simulink model "Transm_Ptbs_V1_MkSfunc"  (R2018b)
settings: Solver=ode3  StartTime=0.0  StopTime=660  FixedStep=0.001  RelTol=1e-3
PreLoadFcn:
  | Transm_Ptbs_V1_BusInfo
model workspace (MAT data in the model file):
  DiffRatio = 3.421
  EV_current = 200
  EV_motion = [20 4 0.8]
  EV_sf = 2000
  EngDriveRatio = 0.813008130081
  Fs = 0
  Fv = 0.0025
  Jcomp = 0.0227
  Jengine = 0.22
  Ki = 251.3274
  Kisa = 346.6583
  Kp_d = 0.47149
  Kp_q = 0.52125
  Ksa = 85.4316
  Ksf = 1996.2651
  Ld = 0.0003752
  Ldq = [0.0003752 0.0004148]
  Lq = 0.0004148
  Mechanical = [0.0227 0.0025 0]
  MotGbRatio = 1
  P = 4
  PolePairs = 4
  RWheel = 0.3
  Rs = 0.2
  T_max = 120
  T_mtpa = [0 13.3131834767 26.6278836885 39.9456159322 53.2678926341 66.5962219318 79.9321062746 93.277041051 106.632513247 120.000000141]
  b_axle = Simulink.Parameter
  b_axle.Value = 10
  b_axle.DataType = 'auto'
  b_axle.Dimensions = [1 1]
  b_driveshaft = Simulink.Parameter
  b_driveshaft.Value = 10
  b_driveshaft.DataType = 'auto'
  b_driveshaft.Dimensions = [1 1]
  ba = 3.4029
  id_mtpa = [0 -0.114523352646 -0.457989076459 -1.03008464374 -1.83029075221 -2.85788367342 -4.11193850568 -5.59133329791 -7.29475400168 -9.22070020138]
  idq0 = [0 0]
  idq_limits = [-9.220699542 166.993501392 167.247872355]
  iq_mtpa = [0 18.5827440345 37.1633719111 55.7397734896 74.3098506185 92.871523015 111.422734008 129.961456105 148.485696337 166.993501356]
  k_axle = Simulink.Parameter
  k_axle.Value = 5000
  k_axle.DataType = 'auto'
  k_axle.Dimensions = [1 1]
  k_driveshaft = Simulink.Parameter
  k_driveshaft.Value = 1000
  k_driveshaft.DataType = 'auto'
  k_driveshaft.Dimensions = [1 1]
  lambda_pm = 0.1194
  mechanical = [0.0227 0.0025 0]
  mot.max_trq = 307
  mot.max_pwr = 124
  mot.spd = [0 500 1000 1500 2000 2500 3000 3500 3857.04487493 4000 4500 5000 5500 6000 6500 7000 7500 8000 8500 9000 9500 10000 10500 11000 11500 12000 12500]
  mot.trq = [307 307 307 307 307 307 307 307 307 296.028194151 263.136172579 236.822555321 215.29323211 197.352129434 182.171196401 169.158968086 157.881703547 148.014097075 139.307385483 131.568086289 124.643450169 118.41127766 112.772645391 107.646616055 102.9663284 98.676064717 94.7290221283]
  mot.trq_cp = [296.028194151 263.136172579 236.822555321 215.29323211 197.352129434 182.171196401 169.158968086 157.881703547 148.014097075 139.307385483 131.568086289 124.643450169 118.41127766 112.772645391 107.646616055 102.9663284 98.676064717 94.7290221283]
  mot.J = 0.02
  mot.damp = 0.0001
  mot.Tc = 0.0267
  mot.map.spdindex = [0 1000 2000 3000 3857 4000 5000 6000 7000 8000 9000 10000 11000 12000 12584]
  mot.map.trqindex = [10 25 50 75 100 125 150 175 200 225 250 275 300 307]
  mot.map.eff = [84  90  90  90  90  90  90  90  90  90  90  90  90  90  90; 84  90  93  95  95  95  96  95  95  95  95  93  93  93  93; 84  90  93  95  95  95  96  95  96  95  95  95  95  93  93; 84  90  93  95  95  95  96  96  96  95  95  95  95  93  93; 84  90  93  95  95  95  96  96  96  95  95  93  93  93  90; 84  88  90  93  93  95  95  96  95  95  95  93  93  93  90; 84  88  90  90  90  93  95  95  95  93  93  93  93  93  90; 84  88  90  90  90  90  93  93  93  93  93  93  93  93  90; 84  84  88  90  90  90  93  93  93  93  93  93  93  93  90; 84  84  88  90  90  90  90  93  93  93  93  93  93  93  90; 84  84  84  90  90  90  90  93  93  93  93  93  93  93  90; 84  84  84  88  90  90  90  93  93  93  93  93  93  93  90; 84  84  84  88  88  88  90  93  93  93  93  93  93  93  90; 84  84  84  88  88  88  90  93  93  93  93  93  93  93  90]
  mot.m = 30
  mot.Cp = 200
  omega_init = 0
  theta_init = 0
  wc_shaft = Simulink.Parameter
  wc_shaft.Value = 0.1
  wc_shaft.DataType = 'auto'
  wc_shaft.Dimensions = [1 1]
libraries: autolibtransamt x1
settings Model: Creator=IAEC Nishito  LastModifiedBy=E00026
settings ConfigSet: Description=|
  | プラント、トップモデル用Configurationパラメータ
  | MILS用　固定ステップ
  | Vehicle Network toolbox のCAN通信を、Simulink Desktop Real timeでリアルタイム動作する
settings DataIOCC: SaveFormat=Array  SaveOutput=off  SignalLogging=off  DSMLogging=off  SaveTime=off
settings OptimizationCC: EfficientMapNaN2IntZero=off
settings DebuggingCC: AlgebraicLoopMsg=error  StateNameClashWarn=warning  SFUnexpectedBacktrackingDiag=warning  SFNoUnconditionalDefaultTransitionDiag=warning  SFExecutionAtInitializationDiag=none
settings HardwareCC: ProdBitPerPointer=32  ProdBitPerSizeT=32  ProdBitPerPtrDiffT=32  ProdLargestAtomicFloat=None  ProdIntDivRoundTo=Undefined  ProdEndianess=Unspecified  ProdWordSize=32  ProdHWDeviceType=32-bit Generic  TargetBitPerPointer=64  TargetBitPerSizeT=64  TargetBitPerPtrDiffT=64  TargetLongLongMode=on  TargetIntDivRoundTo=Zero  TargetEndianess=LittleEndian  TargetWordSize=64  TargetHWDeviceType=MATLAB Host  ProdEqTarget=off
settings ModelReferenceCC: PropagateSignalLabelsOutOfModel=off
settings SFSimCC: SimUseLocalCustomCode=off
settings RTWCC: SystemTargetFile=rtwsfcn.tlc  TemplateMakefile=rtwsfcn_default_tmf  Description=S-Function Target  RTWUseLocalCustomCode=off
settings CodeAppCC: MaxIdLength=128
settings STFCustomTargetCC: ModelReferenceCompliant=off  CompOptLevelCompliant=on  MATLABClassNameForMDSCustomization=Simulink.SoftwareTarget.TargetSpecificTriggerConfigurationBase  GRTInterface=on  SystemTargetFile=rtwsfcn.tlc

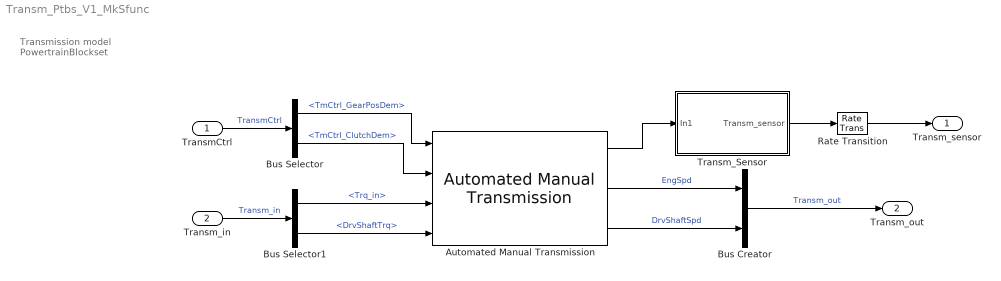
== system Transm_Ptbs_V1_MkSfunc ==
  note: Transmission model
      | PowertrainBlockset
  TransmCtrl : Inport  OutDataTypeStr=Bus: TransmCtrl_Bus  SampleTime=0.001
      settings: AttributesFormatString=|
      | %<OutDataTypeStr>
      | <SampleTime=%<SampleTime>>
  Transm_in : Inport  Port=2  OutDataTypeStr=Bus: Transm_in_Bus  SampleTime=0
      settings: AttributesFormatString=%<OutDataTypeStr>
  Automated Manual Transmission : autolibtransamt/Automated Manual Transmission  VariantControl=0  cntrlType=External control  TransEffModelPopup=Gear only  Jin=.3  bin=.03  omegain_o=0  G=[-1, 0, 1, 2, 3, 4, 5]  Trq_bpts=[25, 50, 75, 100, 150, 200, 250]  omega_bpts=[52.4 78.5 105 131 157 183 209 262 314 419 524]  Temp_bpts=[313 358]  N=[-4.47 ,1, 4.47, 2.47, 1.47, 1, 0.8]  Jout=[0.128 0.01 0.128 0.1 0.062 0.028 0.01]  bout=[.003 .001 .003 .0025 .002 .001 .001]  eta=[0.9, 0.9, 0.9, 0.9, 0.9, 0.95, 0.95]  eta_tbl=reshape([0.53 0.71 0.77 0.79 0.82 0.82 0.82 0.5 0.7 0.77 0.79 0.82 0.82 0.82 0.54 0.72 0.78 0.81 0.83 0.82 0.82 0.56 0.73 0.79 0.81 0.84 0.82 0.82 0.58 0.74 0.79 0.82 0.84 0.82 0.82 0.57 0.74 0.79 0.82 0.84 0.82 0.82 0.58 0.74 0.79 0.82 0.84 0.82 0.82 0.58 0.74 0.79 0.82 0.84 0.82 0.82 0.57 0.74 0.8 0.82 0.85 0.82 0.82 0.55 0.73 0.78 0.81 0.84 0.82 0.82 0.51 0.71 0.77 0.81 0.84 0.82 0.82 0.53 0.71 0.77 0.79 0.82 0.82 0.82 0.5 0.7 0.77 0.79 0.82 0.82 0.82 0.54 0.72 0.78 0.81 0.83 0.82 0.82 0.56 0.73 0.79 0.81 0.84 0.82 0.82 0.58 0.74 0.79 0.82 0.84 0.82 0.82 0.57 0.74 0.79 0.82 0.84 0.82 0.82 0.58 0.74 0.79 0.82 0.84 0.82 0.82 0.58 0.74 0.79 0.82 0.84 0.82 0.82 0.57 0.74 0.8 0.82 0.85 0.82 0.82 0.55 0.73 0.78 0.81 0.84 0.82 0.82 0.51 0.71 0.77 0.81 0.84 0.82 0.82 0.53 0.71 0.77 0.79 0.82 0.82 0.82 0.5 0.7 0.77 0.79 0.82 0.82 0.82 0.54 0.72 0.78 0.81 0.83 0.82 0.82 0.56 0.73 0.79 0.81 0.84 0.82 0.82 0.58 0.74 0.79 0.82 0.84 0.82 0.82 0.57 0.74 0.79 0.82 0.84 0.82 0.82 0.58 0.74 0.79 0.82 0.84 0.82 0.82 0.58 0.74 0.79 0.82 0.84 0.82 0.82 0.57 0.74 0.8 0.82 0.85 0.82 0.82 0.55 0.73 0.78 0.81 0.84 0.82 0.82 0.51 0.71 0.77 0.81 0.84 0.82 0.82 0.7 0.79 0.82 0.83 0.84 0.84 0.84 0.63 0.76 0.8 0.82 0.83 0.84 0.84 0.58 0.74 0.79 0.81 0.83 0.84 0.84 0.58 0.74 0.79 0.81 0.83 0.84 0.84 0.58 0.74 0.79 0.81 0.84 0.84 0.84 0.57 0.73 0.78 0.81 0.84 0.85 0.84 0.57 0.73 0.79 0.81 0.84 0.85 0.84 0.56 0.73 0.78 0.81 0.83 0.85 0.84 0.55 0.73 0.78 0.81 0.84 0.85 0.84 0.52 0.71 0.77 0.8 0.83 0.85 0.84 0.48 0.69 0.76 0.79 0.83 0.84 0.84 0.64 0.76 0.8 0.81 0.83 0.84 0.84 0.56 0.73 0.78 0.8 0.83 0.84 0.84 0.54 0.71 0.77 0.8 0.82 0.84 0.84 0.53 0.71 0.77 0.8 0.83 0.84 0.84 0.51 0.71 0.77 0.8 0.83 0.84 0.85 0.52 0.7 0.77 0.8 0.83 0.84 0.85 0.51 0.71 0.76 0.79 0.83 0.84 0.85 0.5 0.69 0.76 0.79 0.82 0.84 0.85 0.45 0.68 0.75 0.78 0.82 0.84 0.85 0.43 0.67 0.74 0.78 0.81 0.83 0.84 0.38 0.63 0.71 0.75 0.8 0.82 0.83 0.65 0.79 0.84 0.85 0.88 0.89 0.89 0.56 0.75 0.81 0.83 0.86 0.88 0.89 0.52 0.72 0.79 0.83 0.86 0.88 0.88 0.51 0.72 0.79 0.83 0.86 0.88 0.89 0.49 0.71 0.78 0.82 0.86 0.88 0.89 0.47 0.7 0.78 0.82 0.86 0.87 0.88 0.45 0.69 0.77 0.81 0.85 0.87 0.88 0.4 0.67 0.75 0.8 0.84 0.86 0.88 0.3 0.64 0.73 0.78 0.83 0.86 0.87 0.17 0.55 0.67 0.73 0.8 0.83 0.85 0.089 0.45 0.61 0.69 0.77 0.81 0.83 0.61 0.75 0.82 0.84 0.87 0.87 0.88 0.54 0.73 0.8 0.82 0.86 0.87 0.88 0.51 0.71 0.79 0.82 0.86 0.87 0.88 0.52 0.72 0.79 0.82 0.86 0.87 0.89 0.52 0.72 0.8 0.83 0.86 0.88 0.89 0.53 0.72 0.79 0.82 0.86 0.87 0.89 0.5 0.7 0.78 0.82 0.86 0.88 0.88 0.46 0.69 0.77 0.81 0.85 0.87 0.88 0.4 0.67 0.75 0.8 0.83 0.86 0.88 0.33 0.64 0.73 0.78 0.83 0.85 0.87 0.33 0.64 0.73 0.78 0.83 0.85 0.87 0.78 0.85 0.87 0.88 0.89 0.89 0.89 0.73 0.83 0.86 0.88 0.89 0.89 0.89 0.72 0.83 0.86 0.88 0.89 0.89 0.89 0.72 0.83 0.87 0.89 0.9 0.89 0.89 0.72 0.83 0.87 0.88 0.9 0.89 0.89 0.71 0.83 0.87 0.88 0.9 0.89 0.89 0.71 0.83 0.86 0.88 0.9 0.89 0.89 0.7 0.82 0.86 0.88 0.9 0.89 0.89 0.69 0.82 0.86 0.88 0.9 0.89 0.89 0.67 0.81 0.86 0.88 0.9 0.89 0.89 0.63 0.79 0.85 0.87 0.89 0.89 0.89 0.78 0.85 0.87 0.88 0.89 0.89 0.89 0.73 0.83 0.86 0.88 0.89 0.89 0.89 0.72 0.83 0.86 0.88 0.89 0.89 0.89 0.72 0.83 0.87 0.89 0.9 0.89 0.89 0.72 0.83 0.87 0.88 0.9 0.89 0.89 0.71 0.83 0.87 0.88 0.9 0.89 0.89 0.71 0.83 0.86 0.88 0.9 0.89 0.89 0.7 0.82 0.86 0.88 0.9 0.89 0.89 0.69 0.82 0.86 0.88 0.9 0.89 0.89 0.67 0.81 0.86 0.88 0.9 0.89 0.89 0.63 0.79 0.85 0.87 0.89 0.89 0.89 0.78 0.85 0.87 0.88 0.89 0.89 0.89 0.73 0.83 0.86 0.88 0.89 0.89 0.89 0.72 0.83 0.86 0.88 0.89 0.89 0.89 0.72 0.83 0.87 0.89 0.9 0.89 0.89 0.72 0.83 0.87 0.88 0.9 0.89 0.89 0.71 0.83 0.87 0.88 0.9 0.89 0.89 0.71 0.83 0.86 0.88 0.9 0.89 0.89 0.7 0.82 0.86 0.88 0.9 0.89 0.89 0.69 0.82 0.86 0.88 0.9 0.89 0.89 0.67 0.81 0.86 0.88 0.9 0.89 0.89 0.63 0.79 0.85 0.87 0.89 0.89 0.89 0.82 0.87 0.88 0.89 0.89 0.89 0.89 0.81 0.87 0.89 0.89 0.9 0.9 0.89 0.76 0.85 0.87 0.89 0.9 0.89 0.89 0.72 0.83 0.86 0.88 0.89 0.89 0.89 0.72 0.83 0.86 0.88 0.89 0.9 0.89 0.71 0.82 0.86 0.88 0.89 0.9 ...(+1314 chars))  omegaout_o=0  G_o=0  tauc=.02  ts=.15  tc=0.25  R=.2  K_c=5e3  mus=0.6  muk=0.4  ClutchLocked=off  SynchLocked=off  maxAbsSpd=5e3
      settings: SourceProductName=Powertrain Blockset  SourceProductBaseCode=PW
  Bus Creator : BusCreator  Inputs=2  OutDataTypeStr=Bus: Transm_out_Bus
      settings: AttributesFormatString=%<OutDataTypeStr>
  Bus Selector : BusSelector  OutputSignals=TmCtrl_GearPosDem,TmCtrl_ClutchDem
  Bus Selector1 : BusSelector  OutputSignals=Trq_in,DrvShaftTrq
  Rate Transition : RateTransition  Deterministic=off
  Transm_Sensor : Subsystem
  Transm_sensor : Outport  OutDataTypeStr=Bus: Transm_sensor_Bus
      settings: AttributesFormatString=%<OutDataTypeStr>
  Transm_out : Outport  Port=2  OutDataTypeStr=Bus: Transm_out_Bus
      settings: AttributesFormatString=%<OutDataTypeStr>
  wires:
  Automated Manual Transmission/3 -> Bus Creator/2  "DrvShaftSpd"
  TransmCtrl/1 -> Bus Selector/1  "TransmCtrl"
  Bus Selector/1 -> Automated Manual Transmission/1  "<TmCtrl_GearPosDem>"
  Bus Selector/2 -> Automated Manual Transmission/2  "<TmCtrl_ClutchDem>"
  Automated Manual Transmission/2 -> Bus Creator/1  "EngSpd"
  Automated Manual Transmission/1 -> Transm_Sensor/1(In1)
  Transm_Sensor/1(Transm_sensor) -> Rate Transition/1
  Bus Creator/1 -> Transm_out/1  "Transm_out"
  Transm_in/1 -> Bus Selector1/1  "Transm_in"
  Bus Selector1/1 -> Automated Manual Transmission/3  "<Trq_in>"
  Bus Selector1/2 -> Automated Manual Transmission/4  "<DrvShaftTrq>"
  Rate Transition/1 -> Transm_sensor/1

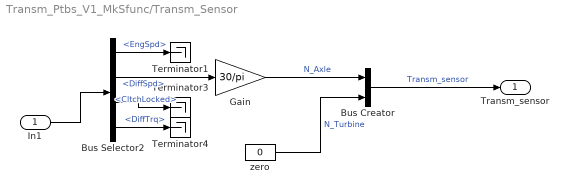
== system Transm_Ptbs_V1_MkSfunc/Transm_Sensor ==
  In1 : Inport
  Bus Creator : BusCreator  Inputs=2  OutDataTypeStr=Bus: Transm_sensor_Bus
      settings: AttributesFormatString=%<OutDataTypeStr>
  Bus Selector2 : BusSelector  OutputSignals=Eng.EngSpd,Diff.DiffSpd,Cltch.CltchLocked,Diff.DiffTrq
  Gain : Gain  Gain=30/pi
  Terminator1 : Terminator
  Terminator3 : Terminator
  Terminator4 : Terminator
  zero : Constant  Value=0
  Transm_sensor : Outport
  wires:
  Bus Creator/1 -> Transm_sensor/1  "Transm_sensor"
  Bus Selector2/4 -> Terminator4/1  "<DiffTrq>"
  Bus Selector2/3 -> Terminator3/1  "<CltchLocked>"
  In1/1 -> Bus Selector2/1
  Gain/1 -> Bus Creator/1  "N_Axle"
  zero/1 -> Bus Creator/2  "N_Turbine"
  Bus Selector2/1 -> Terminator1/1  "<EngSpd>"
  Bus Selector2/2 -> Gain/1  "<DiffSpd>"
